simulink model "fuzzPIK"  (R2021b)
settings: Solver=VariableStepAuto  StartTime=0.0  StopTime=50.0  RelTol=1e-3
libraries: fuzblock x1
settings Model: LastModifiedBy=Tudi
settings OptimizationCC: BlockReduction=off  BooleanDataType=off
settings DebuggingCC: SaveWithParameterizedLinksMsg=none  UnderspecifiedInitializationDetection=Classic  MergeDetectMultiDrivingBlocksExec=none  SignalResolutionControl=TryResolveAllWithWarning
settings HardwareCC: TargetUnknown=on
settings ModelReferenceCC: PropagateSignalLabelsOutOfModel=off

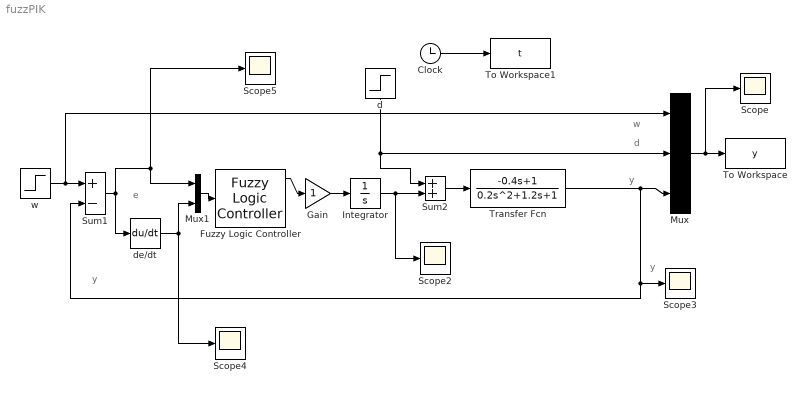
== system fuzzPIK ==
  note: y
  note: w
  note: d
  note: y
  note: e
  note: y
  Clock : Clock
  Fuzzy Logic Controller : fuzblock/Fuzzy Logic  Controller  FIS='tipper.fis'  OutputSampleNumber=101  DataType=double  FuzzifiedInputs=on  RuleFiringStrengths=on  RuleOutputs=on  AggregatedOutputs=on  SimulateUsing=Interpreted execution  OutOfRangeInputValueMessage=warning  NoRuleFiredMessage=warning  EmptyOutputFuzzySetMessage=warning
  Gain : Gain  SaturateOnIntegerOverflow=on
  Integrator : Integrator
  Mux : Mux  Inputs=3
  Mux1 : Mux  Inputs=2
  Scope{,2..5} (5 alike) : Scope
  Sum1 : Sum  Inputs=+-  SaturateOnIntegerOverflow=on
  Sum2 : Sum  SaturateOnIntegerOverflow=on
  To Workspace : ToWorkspace  VariableName=y  SampleTime=-1
  To Workspace1 : ToWorkspace  VariableName=t  SampleTime=-1
  Transfer Fcn : TransferFcn  Numerator=[-0.4 1 ]  Denominator="[0.2  1.2  1]"
  d : Step  Time=5  SampleTime=2
  de/dt : Derivative
  w : Step  Time=2  After=4  SampleTime=1
  wires:
  Sum2/1 -> Transfer Fcn/1
  Clock/1 -> To Workspace1/1
  d/1 -> Sum2/1, Mux/2
  Mux/1 -> To Workspace/1, Scope/1
  w/1 -> Sum1/1, Mux/1
  Sum1/1 -> de/dt/1, Mux1/1, Scope5/1
  Gain/1 -> Integrator/1
  Transfer Fcn/1 -> Mux/3, Scope3/1, Sum1/2
  Integrator/1 -> Sum2/2, Scope2/1
  de/dt/1 -> Mux1/2, Scope4/1
  Mux1/1 -> Fuzzy Logic Controller/1
  Fuzzy Logic Controller/1 -> Gain/1
